simulink model "latlonblk"  (R2019a)
settings: Solver=ode15s  StartTime=0.0  StopTime=10.0  MaxStep=0.01  RelTol=1e-3  EnableMultiTasking=on
settings Model: Creator=Administrator  LastModifiedBy=SomefunAgba
settings DataIOCC: LimitDataPoints=on  SaveFormat=Array
settings OptimizationCC: LifeSpan=inf
settings DebuggingCC: SFUnexpectedBacktrackingDiag=warning  SFNoUnconditionalDefaultTransitionDiag=warning  SFExecutionAtInitializationDiag=none  ArithmeticOperatorsInVariantConditions=warning
settings HardwareCC: ProdBitPerPointer=32  ProdBitPerSizeT=32  ProdBitPerPtrDiffT=32  ProdLargestAtomicFloat=None  ProdIntDivRoundTo=Undefined  ProdEndianess=Unspecified  ProdWordSize=32  ProdHWDeviceType=32-bit Generic
settings ModelReferenceCC: PropagateSignalLabelsOutOfModel=off
settings SFSimCC: SimUseLocalCustomCode=off
settings RTWCC: RTWUseLocalCustomCode=off
settings CodeAppCC: StateflowObjectComments=on
settings GRTTargetCC: TargetLangStandard=C89/C90 (ANSI)  GeneratePreprocessorConditionals=Disable all
settings ConfigComp: CovMetricSettings=dw  CovHtmlReporting=on  CovSaveCumulativeToWorkspaceVar=on  CovSaveSingleToWorkspaceVar=on  CovExternalEMLEnable=off

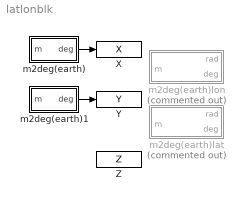
== system latlonblk ==
  X : ToWorkspace  VariableName=X  SampleTime=-1
  Y : ToWorkspace  VariableName=Y  SampleTime=-1
  Z : ToWorkspace  VariableName=Z  SampleTime=-1
  m2deg(earth) : Subsystem
  m2deg(earth)1 : Subsystem
  m2deg(earth)lat : Subsystem  Commented=on
  m2deg(earth)lon : Subsystem  Commented=on
  wires:
  ? -> Z/1  "z"
  ? -> m2deg(earth)1/1(m)  "y"
  ? -> m2deg(earth)/1(m)  "x"
  m2deg(earth)/1(deg) -> X/1
  m2deg(earth)1/1(deg) -> Y/1

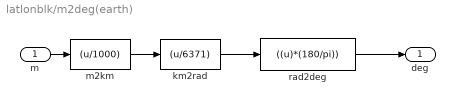
== system latlonblk/m2deg(earth) ==
  m : Inport
  km2rad : Fcn  Expr=(u/6371)
  m2km : Fcn  Expr=(u/1000)
  rad2deg : Fcn  Expr=((u)*(180/pi))
  deg : Outport
  wires:
  m2km/1 -> km2rad/1
  m/1 -> m2km/1
  km2rad/1 -> rad2deg/1
  rad2deg/1 -> deg/1

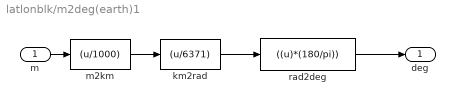
== system latlonblk/m2deg(earth)1 ==
  m : Inport
  km2rad : Fcn  Expr=(u/6371)
  m2km : Fcn  Expr=(u/1000)
  rad2deg : Fcn  Expr=((u)*(180/pi))
  deg : Outport
  wires:
  rad2deg/1 -> deg/1
  km2rad/1 -> rad2deg/1
  m/1 -> m2km/1
  m2km/1 -> km2rad/1

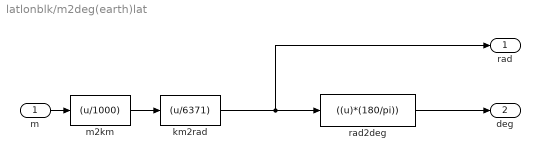
== system latlonblk/m2deg(earth)lat ==
  m : Inport
  km2rad : Fcn  Expr=(u/6371)
  m2km : Fcn  Expr=(u/1000)
  rad2deg : Fcn  Expr=((u)*(180/pi))
  rad : Outport
  deg : Outport  Port=2
  wires:
  m2km/1 -> km2rad/1
  m/1 -> m2km/1
  km2rad/1 -> rad/1, rad2deg/1
  rad2deg/1 -> deg/1

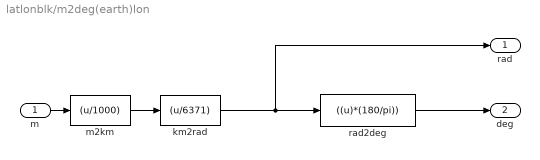
== system latlonblk/m2deg(earth)lon ==
  m : Inport
  km2rad : Fcn  Expr=(u/6371)
  m2km : Fcn  Expr=(u/1000)
  rad2deg : Fcn  Expr=((u)*(180/pi))
  rad : Outport
  deg : Outport  Port=2
  wires:
  rad2deg/1 -> deg/1
  km2rad/1 -> rad2deg/1, rad/1
  m/1 -> m2km/1
  m2km/1 -> km2rad/1
